simulink model "Traffic_light"  (R2024b)
settings: Solver=VariableStepAuto  StartTime=0.0  StopTime=inf  RelTol=1e-3
settings Model: Creator=rohan  LastModifiedBy=rohan

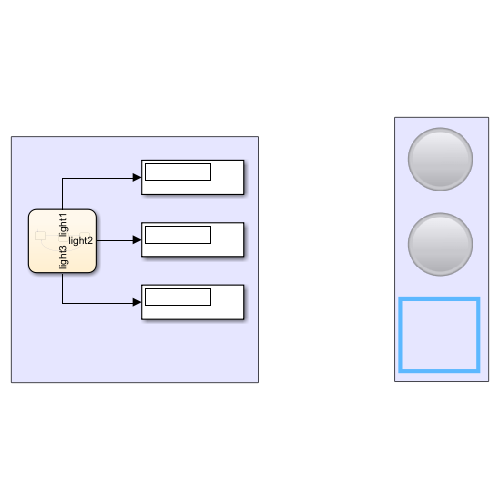
[thumbnail: Simulink's stored preview of the top-level diagram]
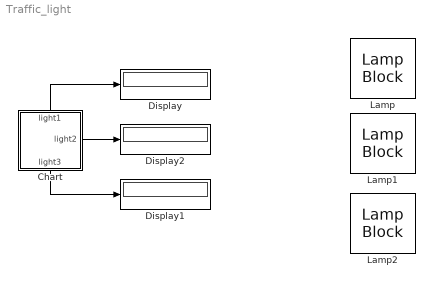
== system Traffic_light ==
  Chart : Stateflow chart  TreatAsAtomicUnit=on
      settings: PortSchema="{\"entries\":[{\"content\":{\"sides\":[{\"content\":{},\"type\":\"ConnectorPlacement.EquallySpacedRectSide\",\"uuid\":\"c92618d2-1111-408a-9f09-ee843f1afcf6\"},{\"content\":{\"connectorIds\":[\"Out3\"],\"side\":\"RIGHT\"},\"type\":\"ConnectorPlacement.EquallySpacedRectSide\",\"uuid\":\"4ea6a14a-f0a6-4323-b1ee-149aaa0777a6\"},{\"content\":{\"connectorIds\":[\"Out1\"],\"side\":\"TOP\"},\"type\":\"ConnectorPlacement.EquallySpacedRectSide\",\"uuid\":\"d35b72d1-fad4-4df8-9ca4-29cdf5e0900d\"},{\"content\":{\"connectorIds\":[\"Out2\"],\"side\":\"BOTTOM\"},\"type\":\"ConnectorPlacement.EquallySpacedRectSide\",\"uuid\":\"05fea230-bb38-4bad-af92-fdb44cc349d8\"}]},\"type\":\"ConnectorPlacement.EquallySpacedConnector\",\"uuid\":\"95e673f6-c33f-4301-8336-52bc3f30fb82\"}],\"packageUris\":[\"http://schema.mathworks.com/mf0/Connector/R2020b\"],\"version\":\"1.0\"}"
  Display : Display
  Display1 : Display
  Display2 : Display
  Lamp : LampBlock  LabelPosition=Hide
  Lamp1 : LampBlock  LabelPosition=Hide
  Lamp2 : LampBlock  LabelPosition=Hide
  wires:
  Chart/2(light3) -> Display1/1
  Chart/1(light1) -> Display/1
  Chart/3(light2) -> Display2/1

== stateflow chart Traffic_light/Chart ==
  state RED
    entry:
    light3=0
    during:
    light1=1
  state YELLOW
    entry:
    light1=0
    during:
    light2=1
  state GREEN
    entry:
    light2=0
    during:
    light3=1
  (default) -> RED
  RED -> YELLOW : after(30,sec)
  YELLOW -> GREEN : after(5,sec)
  GREEN -> RED : after(45,sec)
  data: light1 output; light3 output; light2 output
